simulink model "Force_damper_mass"  (R2018a)
settings: Solver=VariableStepAuto  StartTime=0.0  StopTime=80  RelTol=1e-3
values from neighbouring files (symbols this model uses):
  b = randi([0,1],100,1)    [BPSK.m]    (also in Control_lab2_1.m = [6 0 1]; ShiftKeying_1.m)
  m = sin(2*3.14*t)    [Digital_Lab2.m]    (also in Digital_Lab2_ALaw.m = t.^3)
undefined symbols (not defined in the file or in its folder): k
settings Model: Creator=bhanubhandari  LastModifiedBy=bhanubhandari

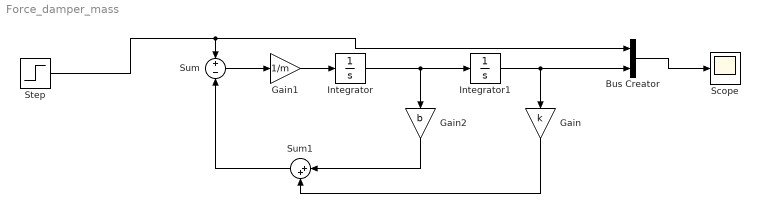
== system Force_damper_mass ==
  Bus Creator : BusCreator  Inputs=2
  Gain : Gain  Gain=k
  Gain1 : Gain  Gain=1/m
  Gain2 : Gain  Gain=b
  Integrator : Integrator
  Integrator1 : Integrator
  Scope : Scope
  Step : Step  SampleTime=0
  Sum : Sum  Inputs=+-
  Sum1 : Sum  Inputs=|++
  wires:
  Sum/1 -> Gain1/1
  Gain1/1 -> Integrator/1
  Integrator/1 -> Integrator1/1, Gain2/1
  Integrator1/1 -> Bus Creator/2, Gain/1
  Gain/1 -> Sum1/2
  Gain2/1 -> Sum1/1
  Sum1/1 -> Sum/2
  Bus Creator/1 -> Scope/1
  Step/1 -> Sum/1, Bus Creator/1
